simulink model "aerotest"  (R2021b)
settings: Solver=VariableStepAuto  StartTime=0.0  StopTime=10.0  RelTol=1e-3
undefined symbols (not defined in the file or in its folder): admireDB
libraries: simulink_extras x103, simulink x24, aerolibatmos2 x1
(part 10 of 13)

== system aerotest/RollMomentCoefficient/MachRegion1/Crmbeta/Crmbeta_ ==
  angleOfSideslip_deg : Inport
  angleOfAttack_deg : Inport  Port=2
  qacorr : Inport  Port=3
  mach_nd : Inport  Port=4
  Abs : Abs
  CRMBAL_BETA_ALFA : Lookup_n-D  BreakpointsForDimension1=admireDB.aerodata_asym_ext.CRMBAL.breakpoints.ALFA  BreakpointsForDimension2=admireDB.aerodata_asym_ext.CRMBAL.breakpoints.BETA  BreakpointsForDimension3=[5, 7]  Table=admireDB.aerodata_asym_ext.CRMBAL.newTable  ExtrapMethod=Clip  InternalRulePriority=Speed  RndMeth=Simplest  InputSameDT=on
      settings: InputPortMap=u0,u1
  CRMEB_QA_M : Lookup_n-D  BreakpointsForDimension1=admireDB.aerodata_asym_ext.CRMEB.breakpoints.M  BreakpointsForDimension2=admireDB.aerodata_asym_ext.CRMEB.breakpoints.QA  BreakpointsForDimension3=[5, 7]  Table=admireDB.aerodata_asym_ext.CRMEB.newTable  ExtrapMethod=Clip  InternalRulePriority=Speed  RndMeth=Simplest  InputSameDT=on
      settings: InputPortMap=u0,u1
  Degrees to Radians : simulink_extras/Transformations/Degrees to Radians
  Product : Product
  Product1 : Product
  Sign : Signum
  Sum : Sum  Inputs=|++
  Crmbeta : Outport
  wires:
  Sum/1 -> Crmbeta/1
  Product1/1 -> Sum/2
  Degrees to Radians/1 -> Product1/1
  CRMEB_QA_M/1 -> Product1/2
  Product/1 -> Sum/1
  Abs/1 -> CRMBAL_BETA_ALFA/2
  Sign/1 -> Product/1
  CRMBAL_BETA_ALFA/1 -> Product/2
  angleOfSideslip_deg/1 -> Abs/1, Sign/1, Degrees to Radians/1
  mach_nd/1 -> CRMEB_QA_M/1
  angleOfAttack_deg/1 -> CRMBAL_BETA_ALFA/1
  qacorr/1 -> CRMEB_QA_M/2

== system aerotest/RollMomentCoefficient/MachRegion1/Crmbetad/Crmbetad_ ==
  angleOfAttack_deg : Inport
  betad : Inport  Port=2
  CRMBDL_ALFA : Lookup_n-D  NumberOfTableDimensions=1  BreakpointsForDimension1=admireDB.aerodata_asym_ext.CRMBDL.breakpoints.ALFA  BreakpointsForDimension3=[5, 7]  Table=admireDB.aerodata_asym_ext.CRMBDL.newTable  ExtrapMethod=Clip  InternalRulePriority=Speed  RndMeth=Simplest  InputSameDT=on
  Product : Product  Inputs=**
  Crmbetad : Outport
  wires:
  angleOfAttack_deg/1 -> CRMBDL_ALFA/1
  Product/1 -> Crmbetad/1
  CRMBDL_ALFA/1 -> Product/1
  betad/1 -> Product/2

== system aerotest/RollMomentCoefficient/MachRegion1/Crmblg/Crmblg_ ==
  dLG : Inport
  angleOfAttack_deg : Inport  Port=2
  angleOfSideslip_deg : Inport  Port=3
  CRMBLST_NG_DOOR_ALFA : Lookup_n-D  BreakpointsForDimension1=admireDB.aerodata_asym_ext.CRMBLST.breakpoints.ALFA  BreakpointsForDimension2=admireDB.aerodata_asym_ext.CRMBLST.breakpoints.NG_DOOR  BreakpointsForDimension3=[5, 7]  Table=admireDB.aerodata_asym_ext.CRMBLST.newTable  ExtrapMethod=Clip  InternalRulePriority=Speed  RndMeth=Simplest  InputSameDT=on
      settings: InputPortMap=u0,u1
  Degrees to Radians : simulink_extras/Transformations/Degrees to Radians
  Product : Product  Inputs=3
  Crmblg : Outport
  wires:
  Degrees to Radians/1 -> Product/3
  CRMBLST_NG_DOOR_ALFA/1 -> Product/2
  dLG/1 -> CRMBLST_NG_DOOR_ALFA/2, Product/1
  angleOfAttack_deg/1 -> CRMBLST_NG_DOOR_ALFA/1
  Product/1 -> Crmblg/1
  angleOfSideslip_deg/1 -> Degrees to Radians/1

== system aerotest/RollMomentCoefficient/MachRegion1/Crmdai/Crmdai_ ==
  dAI : Inport
  angleOfAttack_deg : Inport  Port=2
  dEI : Inport  Port=3
  eieff : Inport  Port=4
  qacorr : Inport  Port=5
  mach_nd : Inport  Port=6
  Abs : Abs
  CRMDAAL_DA_ALFA : Lookup_n-D  BreakpointsForDimension1=admireDB.aerodata_asym_ext.CRMDAAL.breakpoints.ALFA  BreakpointsForDimension2=admireDB.aerodata_asym_ext.CRMDAAL.breakpoints.DA  BreakpointsForDimension3=[5, 7]  Table=admireDB.aerodata_asym_ext.CRMDAAL.newTable  ExtrapMethod=Clip  InternalRulePriority=Speed  RndMeth=Simplest  InputSameDT=on
      settings: InputPortMap=u0,u1
  CRMDAL_DE_ALFA : Lookup_n-D  BreakpointsForDimension1=admireDB.aerodata_asym_ext.CRMDAL.breakpoints.ALFA  BreakpointsForDimension2=admireDB.aerodata_asym_ext.CRMDAL.breakpoints.DE  BreakpointsForDimension3=[5, 7]  Table=admireDB.aerodata_asym_ext.CRMDAL.newTable  ExtrapMethod=Clip  InternalRulePriority=Speed  RndMeth=Simplest  InputSameDT=on
      settings: InputPortMap=u0,u1
  CRMDAL_DE_ALFA_1 : Lookup_n-D  BreakpointsForDimension1=admireDB.aerodata_asym_ext.CRMDAL.breakpoints.ALFA  BreakpointsForDimension2=admireDB.aerodata_asym_ext.CRMDAL.breakpoints.DE  BreakpointsForDimension3=[5, 7]  Table=admireDB.aerodata_asym_ext.CRMDAL.newTable  ExtrapMethod=Clip  InternalRulePriority=Speed  RndMeth=Simplest  InputSameDT=on
      settings: InputPortMap=u0,u1
  CRMEDAI_QA_M : Lookup_n-D  BreakpointsForDimension1=admireDB.aerodata_asym_ext.CRMEDAI.breakpoints.M  BreakpointsForDimension2=admireDB.aerodata_asym_ext.CRMEDAI.breakpoints.QA  BreakpointsForDimension3=[5, 7]  Table=admireDB.aerodata_asym_ext.CRMEDAI.newTable  ExtrapMethod=Clip  InternalRulePriority=Speed  RndMeth=Simplest  InputSameDT=on
      settings: InputPortMap=u0,u1
  Degrees to Radians : simulink_extras/Transformations/Degrees to Radians
  Product : Product
  Product1 : Product
  Product2 : Product  Inputs=3
  Sign : Signum
  Sum : Sum  Inputs=|+-
  Sum1 : Sum  Inputs=|++
  dE_cnst : Constant  Value=0.0
  Crmdai : Outport
  wires:
  CRMEDAI_QA_M/1 -> Product2/3
  qacorr/1 -> CRMEDAI_QA_M/2
  mach_nd/1 -> CRMEDAI_QA_M/1
  eieff/1 -> Product2/2
  Sum1/1 -> Product2/1
  Product/1 -> Sum1/2
  Product1/1 -> Sum1/1
  Sign/1 -> Product1/1
  CRMDAAL_DA_ALFA/1 -> Product1/2
  Degrees to Radians/1 -> Product/1
  Sum/1 -> Product/2
  CRMDAL_DE_ALFA_1/1 -> Sum/2
  CRMDAL_DE_ALFA/1 -> Sum/1
  dEI/1 -> CRMDAL_DE_ALFA/2
  dE_cnst/1 -> CRMDAL_DE_ALFA_1/2
  dAI/1 -> Abs/1, Sign/1, Degrees to Radians/1
  Abs/1 -> CRMDAAL_DA_ALFA/2
  angleOfAttack_deg/1 -> CRMDAAL_DA_ALFA/1, CRMDAL_DE_ALFA_1/1, CRMDAL_DE_ALFA/1
  Product2/1 -> Crmdai/1

== system aerotest/RollMomentCoefficient/MachRegion1/Crmdaib/Crmdaib_ ==
  angleOfAttack_deg : Inport
  dAI : Inport  Port=2
  angleOfSideslip_deg : Inport  Port=3
  eieff : Inport  Port=4
  Abs : Abs
  Abs1 : Abs
  Abs2 : Abs
  CRMDABAL_ALFA : Lookup_n-D  NumberOfTableDimensions=1  BreakpointsForDimension1=admireDB.aerodata_asym_ext.CRMDABAL.breakpoints.ALFA  BreakpointsForDimension3=[5, 7]  Table=admireDB.aerodata_asym_ext.CRMDABAL.newTable  ExtrapMethod=Clip  InternalRulePriority=Speed  RndMeth=Simplest  InputSameDT=on
  Constant : Constant  Value=30
  Constant1 : Constant  Value=20
  Product : Product  Inputs=**/*/*
  Crmdaib : Outport
  wires:
  eieff/1 -> Product/6
  Abs2/1 -> Product/4
  Constant1/1 -> Product/5
  angleOfSideslip_deg/1 -> Abs2/1
  Constant/1 -> Product/3
  Abs1/1 -> Product/2
  Abs/1 -> CRMDABAL_ALFA/1
  dAI/1 -> Abs1/1
  CRMDABAL_ALFA/1 -> Product/1
  angleOfAttack_deg/1 -> Abs/1
  Product/1 -> Crmdaib/1

== system aerotest/RollMomentCoefficient/MachRegion1/Crmday/Crmday_ ==
  dAY : Inport
  angleOfAttack_deg : Inport  Port=2
  dEY : Inport  Port=3
  eoeff : Inport  Port=4
  qacorr : Inport  Port=5
  mach_nd : Inport  Port=6
  Abs : Abs
  CRMDAAL_DA_ALFA : Lookup_n-D  BreakpointsForDimension1=admireDB.aerodata_asym_ext.CRMDAAL.breakpoints.ALFA  BreakpointsForDimension2=admireDB.aerodata_asym_ext.CRMDAAL.breakpoints.DA  BreakpointsForDimension3=[5, 7]  Table=admireDB.aerodata_asym_ext.CRMDAAL.newTable  ExtrapMethod=Clip  InternalRulePriority=Speed  RndMeth=Simplest  InputSameDT=on
      settings: InputPortMap=u0,u1
  CRMDAL_DE_ALFA : Lookup_n-D  BreakpointsForDimension1=admireDB.aerodata_asym_ext.CRMDAL.breakpoints.ALFA  BreakpointsForDimension2=admireDB.aerodata_asym_ext.CRMDAL.breakpoints.DE  BreakpointsForDimension3=[5, 7]  Table=admireDB.aerodata_asym_ext.CRMDAL.newTable  ExtrapMethod=Clip  InternalRulePriority=Speed  RndMeth=Simplest  InputSameDT=on
      settings: InputPortMap=u0,u1
  CRMDAL_DE_ALFA_1 : Lookup_n-D  BreakpointsForDimension1=admireDB.aerodata_asym_ext.CRMDAL.breakpoints.ALFA  BreakpointsForDimension2=admireDB.aerodata_asym_ext.CRMDAL.breakpoints.DE  BreakpointsForDimension3=[5, 7]  Table=admireDB.aerodata_asym_ext.CRMDAL.newTable  ExtrapMethod=Clip  InternalRulePriority=Speed  RndMeth=Simplest  InputSameDT=on
      settings: InputPortMap=u0,u1
  CRMEDAY_QA_M : Lookup_n-D  BreakpointsForDimension1=admireDB.aerodata_asym_ext.CRMEDAY.breakpoints.M  BreakpointsForDimension2=admireDB.aerodata_asym_ext.CRMEDAY.breakpoints.QA  BreakpointsForDimension3=[5, 7]  Table=admireDB.aerodata_asym_ext.CRMEDAY.newTable  ExtrapMethod=Clip  InternalRulePriority=Speed  RndMeth=Simplest  InputSameDT=on
      settings: InputPortMap=u0,u1
  Degrees to Radians : simulink_extras/Transformations/Degrees to Radians
  Product : Product
  Product1 : Product
  Product2 : Product  Inputs=3
  Sign : Signum
  Sum : Sum  Inputs=|+-
  Sum1 : Sum  Inputs=|++
  dE_cnst : Constant  Value=0.0
  Crmdai : Outport
  wires:
  dE_cnst/1 -> CRMDAL_DE_ALFA_1/2
  Product2/1 -> Crmdai/1
  angleOfAttack_deg/1 -> CRMDAL_DE_ALFA_1/1, CRMDAL_DE_ALFA/1, CRMDAAL_DA_ALFA/1
  Abs/1 -> CRMDAAL_DA_ALFA/2
  dAY/1 -> Abs/1, Sign/1, Degrees to Radians/1
  dEY/1 -> CRMDAL_DE_ALFA/2
  CRMDAL_DE_ALFA/1 -> Sum/1
  CRMDAL_DE_ALFA_1/1 -> Sum/2
  Sum/1 -> Product/2
  Degrees to Radians/1 -> Product/1
  CRMDAAL_DA_ALFA/1 -> Product1/2
  Sign/1 -> Product1/1
  Product1/1 -> Sum1/1
  Product/1 -> Sum1/2
  Sum1/1 -> Product2/1
  eoeff/1 -> Product2/2
  qacorr/1 -> CRMEDAY_QA_M/2
  mach_nd/1 -> CRMEDAY_QA_M/1
  CRMEDAY_QA_M/1 -> Product2/3

== system aerotest/RollMomentCoefficient/MachRegion1/Crmdayb/Crmdaib_ ==
  angleOfAttack_deg : Inport
  dAY : Inport  Port=2
  angleOfSideslip_deg : Inport  Port=3
  eoeff : Inport  Port=4
  Abs : Abs
  Abs1 : Abs
  Abs2 : Abs
  CRMDABAL_ALFA : Lookup_n-D  NumberOfTableDimensions=1  BreakpointsForDimension1=admireDB.aerodata_asym_ext.CRMDABAL.breakpoints.ALFA  BreakpointsForDimension3=[5, 7]  Table=admireDB.aerodata_asym_ext.CRMDABAL.newTable  ExtrapMethod=Clip  InternalRulePriority=Speed  RndMeth=Simplest  InputSameDT=on
  Constant : Constant  Value=30
  Constant1 : Constant  Value=20
  Product : Product  Inputs=**/*/*
  Crmdaib : Outport
  wires:
  Product/1 -> Crmdaib/1
  angleOfAttack_deg/1 -> Abs/1
  CRMDABAL_ALFA/1 -> Product/1
  dAY/1 -> Abs1/1
  Abs/1 -> CRMDABAL_ALFA/1
  Abs1/1 -> Product/2
  Constant/1 -> Product/3
  angleOfSideslip_deg/1 -> Abs2/1
  Constant1/1 -> Product/5
  Abs2/1 -> Product/4
  eoeff/1 -> Product/6

== system aerotest/RollMomentCoefficient/MachRegion1/Crmdna/Crmdna_ ==
  dNE : Inport
  angleOfAttack_deg : Inport  Port=2
  dNA : Inport  Port=3
  CRMDNAAL_DNE_ALFA : Lookup_n-D  BreakpointsForDimension1=admireDB.aerodata_asym_ext.CRMDNAAL.breakpoints.ALFA  BreakpointsForDimension2=admireDB.aerodata_asym_ext.CRMDNAAL.breakpoints.DNE  BreakpointsForDimension3=[5, 7]  Table=admireDB.aerodata_asym_ext.CRMDNAAL.newTable  ExtrapMethod=Clip  InternalRulePriority=Speed  RndMeth=Simplest  InputSameDT=on
      settings: InputPortMap=u0,u1
  Degrees to Radians : simulink_extras/Transformations/Degrees to Radians
  Product : Product  Inputs=**
  Crmdna : Outport
  wires:
  Degrees to Radians/1 -> Product/2
  CRMDNAAL_DNE_ALFA/1 -> Product/1
  dNA/1 -> Degrees to Radians/1
  angleOfAttack_deg/1 -> CRMDNAAL_DNE_ALFA/1
  dNE/1 -> CRMDNAAL_DNE_ALFA/2
  Product/1 -> Crmdna/1

== system aerotest/RollMomentCoefficient/MachRegion1/Crmdr/Crmdr_ ==
  angleOfAttack_deg : Inport
  dR : Inport  Port=2
  angleOfSideslip_deg : Inport  Port=3
  qacorr : Inport  Port=4
  mach_nd : Inport  Port=5
  Abs : Abs
  CRMBDRAL_ALFA_DR_BETA : Lookup_n-D  NumberOfTableDimensions=3  BreakpointsForDimension1=admireDB.aerodata_asym_ext.CRMBDRAL.breakpoints.ALFA  BreakpointsForDimension2=admireDB.aerodata_asym_ext.CRMBDRAL.breakpoints.DR  BreakpointsForDimension3=admireDB.aerodata_asym_ext.CRMBDRAL.breakpoints.BETA  Table=admireDB.aerodata_asym_ext.CRMBDRAL.newTable  ExtrapMethod=Clip  InternalRulePriority=Speed  RndMeth=Simplest  InputSameDT=on
      settings: InputPortMap=u0,u1,u2
  CRMEDR_QA_M : Lookup_n-D  BreakpointsForDimension1=admireDB.aerodata_asym_ext.CRMEDR.breakpoints.M  BreakpointsForDimension2=admireDB.aerodata_asym_ext.CRMEDR.breakpoints.QA  BreakpointsForDimension3=[5, 7]  Table=admireDB.aerodata_asym_ext.CRMEDR.newTable  ExtrapMethod=Clip  InternalRulePriority=Speed  RndMeth=Simplest  InputSameDT=on
      settings: InputPortMap=u0,u1
  Product : Product
  Crmdr : Outport
  wires:
  CRMBDRAL_ALFA_DR_BETA/1 -> Product/1
  CRMEDR_QA_M/1 -> Product/2
  angleOfAttack_deg/1 -> CRMBDRAL_ALFA_DR_BETA/1
  angleOfSideslip_deg/1 -> Abs/1
  dR/1 -> CRMBDRAL_ALFA_DR_BETA/2
  Abs/1 -> CRMBDRAL_ALFA_DR_BETA/3
  qacorr/1 -> CRMEDR_QA_M/2
  mach_nd/1 -> CRMEDR_QA_M/1
  Product/1 -> Crmdr/1

== system aerotest/RollMomentCoefficient/MachRegion1/Crmp/Crmp_ ==
  dN : Inport
  angleOfAttack_deg : Inport  Port=2
  qacorr : Inport  Port=3
  mach_nd : Inport  Port=4
  pc : Inport  Port=5
  CRMEP_QA_M : Lookup_n-D  BreakpointsForDimension1=admireDB.aerodata_asym_ext.CRMEP.breakpoints.M  BreakpointsForDimension2=admireDB.aerodata_asym_ext.CRMEP.breakpoints.QA  BreakpointsForDimension3=[5, 7]  Table=admireDB.aerodata_asym_ext.CRMEP.newTable  ExtrapMethod=Clip  InternalRulePriority=Speed  RndMeth=Simplest  InputSameDT=on
      settings: InputPortMap=u0,u1
  CRMPAL_DN_ALFA : Lookup_n-D  BreakpointsForDimension1=admireDB.aerodata_asym_ext.CRMPAL.breakpoints.ALFA  BreakpointsForDimension2=admireDB.aerodata_asym_ext.CRMPAL.breakpoints.DN  BreakpointsForDimension3=[5, 7]  Table=admireDB.aerodata_asym_ext.CRMPAL.newTable  ExtrapMethod=Clip  InternalRulePriority=Speed  RndMeth=Simplest  InputSameDT=on
      settings: InputPortMap=u0,u1
  Product : Product  Inputs=3
  Crmp : Outport
  wires:
  Product/1 -> Crmp/1
  pc/1 -> Product/2
  CRMEP_QA_M/1 -> Product/3
  CRMPAL_DN_ALFA/1 -> Product/1
  angleOfAttack_deg/1 -> CRMPAL_DN_ALFA/1
  dN/1 -> CRMPAL_DN_ALFA/2
  mach_nd/1 -> CRMEP_QA_M/1
  qacorr/1 -> CRMEP_QA_M/2

== system aerotest/RollMomentCoefficient/MachRegion1/Crmpbeta/Crmpbeta_ ==
  angleOfSideslip_deg : Inport
  angleOfAttack_deg : Inport  Port=2
  pc : Inport  Port=3
  Abs : Abs
  CRMPBA_BETA_ALFA : Lookup_n-D  BreakpointsForDimension1=admireDB.aerodata_asym_ext.CRMPBA.breakpoints.ALFA  BreakpointsForDimension2=admireDB.aerodata_asym_ext.CRMPBA.breakpoints.BETA  BreakpointsForDimension3=[5, 7]  Table=admireDB.aerodata_asym_ext.CRMPBA.newTable  ExtrapMethod=Clip  InternalRulePriority=Speed  RndMeth=Simplest  InputSameDT=on
      settings: InputPortMap=u0,u1
  Product : Product  Inputs=**
  Crmpbeta : Outport
  wires:
  Abs/1 -> CRMPBA_BETA_ALFA/2
  CRMPBA_BETA_ALFA/1 -> Product/1
  angleOfSideslip_deg/1 -> Abs/1
  angleOfAttack_deg/1 -> CRMPBA_BETA_ALFA/1
  pc/1 -> Product/2
  Product/1 -> Crmpbeta/1

== system aerotest/RollMomentCoefficient/MachRegion1/Crmr/Crmr_ ==
  dN : Inport
  angleOfAttack_deg : Inport  Port=2
  rc : Inport  Port=3
  CRMRAL_DN_ALFA : Lookup_n-D  BreakpointsForDimension1=admireDB.aerodata_asym_ext.CRMRAL.breakpoints.ALFA  BreakpointsForDimension2=admireDB.aerodata_asym_ext.CRMRAL.breakpoints.DN  BreakpointsForDimension3=[5, 7]  Table=admireDB.aerodata_asym_ext.CRMRAL.newTable  ExtrapMethod=Clip  InternalRulePriority=Speed  RndMeth=Simplest  InputSameDT=on
      settings: InputPortMap=u0,u1
  Product : Product  Inputs=**
  Crmr : Outport
  wires:
  CRMRAL_DN_ALFA/1 -> Product/1
  angleOfAttack_deg/1 -> CRMRAL_DN_ALFA/1
  dN/1 -> CRMRAL_DN_ALFA/2
  Product/1 -> Crmr/1
  rc/1 -> Product/2

== system aerotest/RollMomentCoefficient/MachRegion1/Crmrbeta/Crmrbeta_ ==
  angleOfSideslip_deg : Inport
  angleOfAttack_deg : Inport  Port=2
  rc : Inport  Port=3
  Abs : Abs
  CRMRBA_BETA_ALFA : Lookup_n-D  BreakpointsForDimension1=admireDB.aerodata_asym_ext.CRMRBA.breakpoints.ALFA  BreakpointsForDimension2=admireDB.aerodata_asym_ext.CRMRBA.breakpoints.BETA  BreakpointsForDimension3=[5, 7]  Table=admireDB.aerodata_asym_ext.CRMRBA.newTable  ExtrapMethod=Clip  InternalRulePriority=Speed  RndMeth=Simplest  InputSameDT=on
      settings: InputPortMap=u0,u1
  Product : Product  Inputs=**
  Crmrbeta : Outport
  wires:
  Abs/1 -> CRMRBA_BETA_ALFA/2
  angleOfSideslip_deg/1 -> Abs/1
  angleOfAttack_deg/1 -> CRMRBA_BETA_ALFA/1
  rc/1 -> Product/2
  Product/1 -> Crmrbeta/1
  CRMRBA_BETA_ALFA/1 -> Product/1

== system aerotest/RollMomentCoefficient/MachRegion1/Crmrde/Crmrde_ ==
  mach_nd : Inport
  angleOfAttack_deg : Inport  Port=2
  rc : Inport  Port=3
  dEI : Inport  Port=4
  eieff : Inport  Port=5
  dey : Inport  Port=6
  eoeff : Inport  Port=7
  CRMRDEM_M : Lookup_n-D  NumberOfTableDimensions=1  BreakpointsForDimension1=admireDB.aerodata_asym_ext.CRMRDEM.breakpoints.M  BreakpointsForDimension3=[5, 7]  Table=admireDB.aerodata_asym_ext.CRMRDEM.newTable  ExtrapMethod=Clip  InternalRulePriority=Speed  RndMeth=Simplest  InputSameDT=on
  CRMRKA_ALFA : Lookup_n-D  NumberOfTableDimensions=1  BreakpointsForDimension1=admireDB.aerodata_asym_ext.CRMRKA.breakpoints.ALFA  BreakpointsForDimension3=[5, 7]  Table=admireDB.aerodata_asym_ext.CRMRKA.newTable  ExtrapMethod=Clip  InternalRulePriority=Speed  RndMeth=Simplest  InputSameDT=on
  Constant : Constant  Value=1/30
  Constant1 : Constant  Value=1/30
  Product : Product  Inputs=****
  Product1 : Product  Inputs=3
  Product2 : Product  Inputs=3
  Sum : Sum  Inputs=|++
  Crmrbeta : Outport
  wires:
  Sum/1 -> Product/4
  Product2/1 -> Sum/2
  Product1/1 -> Sum/1
  dey/1 -> Product2/1
  eoeff/1 -> Product2/3
  Constant1/1 -> Product2/2
  Constant/1 -> Product1/2
  eieff/1 -> Product1/3
  dEI/1 -> Product1/1
  CRMRKA_ALFA/1 -> Product/2
  CRMRDEM_M/1 -> Product/1
  mach_nd/1 -> CRMRDEM_M/1
  angleOfAttack_deg/1 -> CRMRKA_ALFA/1
  Product/1 -> Crmrbeta/1
  rc/1 -> Product/3

== system aerotest/RollMomentCoefficient/MachRegion2/Crmbasic/Crmbasic_ ==
  angleOfAttack_deg : Inport
  tflow : Inport  Port=2
  Abs : Abs
  CRMZERO_ALFA : Lookup_n-D  NumberOfTableDimensions=1  BreakpointsForDimension1=admireDB.aerodata_asym_ext.CRMZERO.breakpoints.ALFA  BreakpointsForDimension3=[5, 7]  Table=admireDB.aerodata_asym_ext.CRMZERO.newTable  ExtrapMethod=Clip  InternalRulePriority=Speed  RndMeth=Simplest  InputSameDT=on
  Product : Product
  Crmbasic : Outport
  wires:
  tflow/1 -> Product/2
  Product/1 -> Crmbasic/1
  CRMZERO_ALFA/1 -> Product/1
  angleOfAttack_deg/1 -> Abs/1
  Abs/1 -> CRMZERO_ALFA/1

== system aerotest/RollMomentCoefficient/MachRegion2/Crmbde/Crmbde_ ==
  angleOfAttack_deg : Inport
  dN : Inport  Port=2
  dEI : Inport  Port=3
  angleOfSideslip_deg : Inport  Port=4
  dEY : Inport  Port=5
  eieff : Inport  Port=6
  eoeff : Inport  Port=7
  Abs : Abs
  CRMDEB_ALFA_DN_DE_BETA : Lookup_n-D  NumberOfTableDimensions=4  BreakpointsForDimension1=admireDB.aerodata_asym_ext.CRMDEB.breakpoints.ALFA  BreakpointsForDimension2=admireDB.aerodata_asym_ext.CRMDEB.breakpoints.DN  BreakpointsForDimension3=admireDB.aerodata_asym_ext.CRMDEB.breakpoints.DE  BreakpointsForDimension4=admireDB.aerodata_asym_ext.CRMDEB.breakpoints.BETA  Table=admireDB.aerodata_asym_ext.CRMDEB.newTable  ExtrapMethod=Clip  InternalRulePriority=Speed  RndMeth=Simplest  InputSameDT=on
      settings: InputPortMap=u0,u1,u2,u3
  CRMDEB_ALFA_DN_DE_BETA1 : Lookup_n-D  NumberOfTableDimensions=4  BreakpointsForDimension1=admireDB.aerodata_asym_ext.CRMDEB.breakpoints.ALFA  BreakpointsForDimension2=admireDB.aerodata_asym_ext.CRMDEB.breakpoints.DN  BreakpointsForDimension3=admireDB.aerodata_asym_ext.CRMDEB.breakpoints.DE  BreakpointsForDimension4=admireDB.aerodata_asym_ext.CRMDEB.breakpoints.BETA  Table=admireDB.aerodata_asym_ext.CRMDEB.newTable  ExtrapMethod=Clip  InternalRulePriority=Speed  RndMeth=Simplest  InputSameDT=on
      settings: InputPortMap=u0,u1,u2,u3
  Product : Product  Inputs=**
  Product1 : Product  Inputs=**
  Product2 : Product
  Sign : Signum
  Sum : Sum  Inputs=|++
  Crmbde : Outport
  wires:
  dEY/1 -> CRMDEB_ALFA_DN_DE_BETA1/3
  dEI/1 -> CRMDEB_ALFA_DN_DE_BETA/3
  dN/1 -> CRMDEB_ALFA_DN_DE_BETA/2, CRMDEB_ALFA_DN_DE_BETA1/2
  angleOfAttack_deg/1 -> CRMDEB_ALFA_DN_DE_BETA/1, CRMDEB_ALFA_DN_DE_BETA1/1
  Abs/1 -> CRMDEB_ALFA_DN_DE_BETA1/4, CRMDEB_ALFA_DN_DE_BETA/4
  angleOfSideslip_deg/1 -> Sign/1, Abs/1
  CRMDEB_ALFA_DN_DE_BETA/1 -> Product/1
  CRMDEB_ALFA_DN_DE_BETA1/1 -> Product1/2
  eieff/1 -> Product/2
  eoeff/1 -> Product1/1
  Sum/1 -> Product2/2
  Product/1 -> Sum/1
  Product1/1 -> Sum/2
  Product2/1 -> Crmbde/1
  Sign/1 -> Product2/1

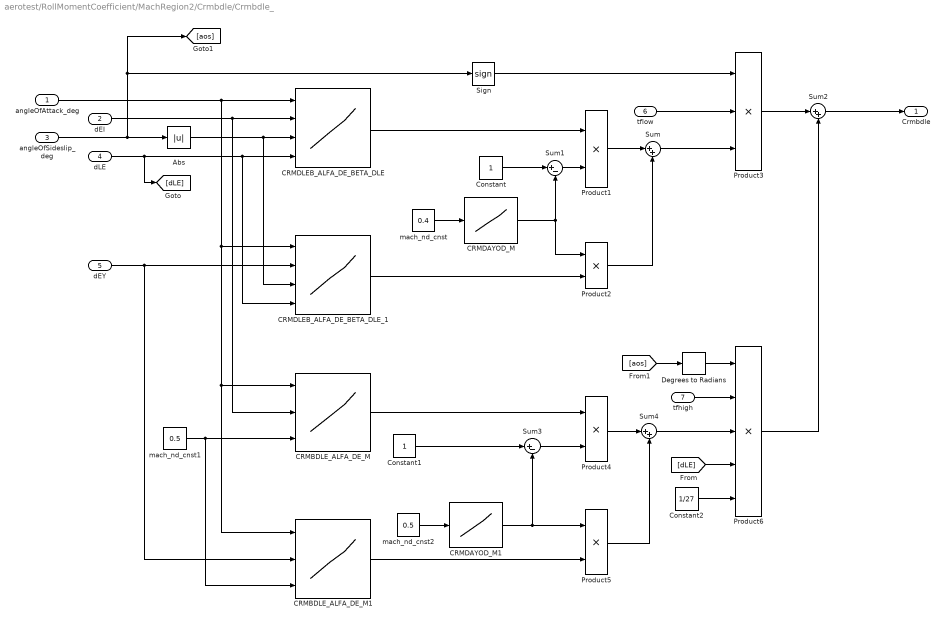
== system aerotest/RollMomentCoefficient/MachRegion2/Crmbdle/Crmbdle_ ==
  angleOfAttack_deg : Inport
  dEI : Inport  Port=2
  angleOfSideslip_deg : Inport  Port=3
  dLE : Inport  Port=4
  dEY : Inport  Port=5
  tflow : Inport  Port=6
  tfhigh : Inport  Port=7
  Abs : Abs
  CRMBDLE_ALFA_DE_M : Lookup_n-D  NumberOfTableDimensions=3  BreakpointsForDimension1=admireDB.aerodata_asym_ext.CRMBDLE.breakpoints.ALFA  BreakpointsForDimension2=admireDB.aerodata_asym_ext.CRMBDLE.breakpoints.DE  BreakpointsForDimension3=admireDB.aerodata_asym_ext.CRMBDLE.breakpoints.M  Table=admireDB.aerodata_asym_ext.CRMBDLE.newTable  ExtrapMethod=Clip  InternalRulePriority=Speed  RndMeth=Simplest  InputSameDT=on
      settings: InputPortMap=u0,u1,u2
  CRMBDLE_ALFA_DE_M1 : Lookup_n-D  NumberOfTableDimensions=3  BreakpointsForDimension1=admireDB.aerodata_asym_ext.CRMBDLE.breakpoints.ALFA  BreakpointsForDimension2=admireDB.aerodata_asym_ext.CRMBDLE.breakpoints.DE  BreakpointsForDimension3=admireDB.aerodata_asym_ext.CRMBDLE.breakpoints.M  Table=admireDB.aerodata_asym_ext.CRMBDLE.newTable  ExtrapMethod=Clip  InternalRulePriority=Speed  RndMeth=Simplest  InputSameDT=on
      settings: InputPortMap=u0,u1,u2
  CRMDAYOD_M : Lookup_n-D  NumberOfTableDimensions=1  BreakpointsForDimension1=admireDB.aerodata_asym_ext.CRMDAYOD.breakpoints.M  BreakpointsForDimension3=[5, 7]  Table=admireDB.aerodata_asym_ext.CRMDAYOD.newTable  ExtrapMethod=Clip  InternalRulePriority=Speed  RndMeth=Simplest  InputSameDT=on
  CRMDAYOD_M1 : Lookup_n-D  NumberOfTableDimensions=1  BreakpointsForDimension1=admireDB.aerodata_asym_ext.CRMDAYOD.breakpoints.M  BreakpointsForDimension3=[5, 7]  Table=admireDB.aerodata_asym_ext.CRMDAYOD.newTable  ExtrapMethod=Clip  InternalRulePriority=Speed  RndMeth=Simplest  InputSameDT=on
  CRMDLEB_ALFA_DE_BETA_DLE : Lookup_n-D  NumberOfTableDimensions=4  BreakpointsForDimension1=admireDB.aerodata_asym_ext.CRMDLEB.breakpoints.ALFA  BreakpointsForDimension2=admireDB.aerodata_asym_ext.CRMDLEB.breakpoints.DE  BreakpointsForDimension3=admireDB.aerodata_asym_ext.CRMDLEB.breakpoints.BETA  BreakpointsForDimension4=admireDB.aerodata_asym_ext.CRMDLEB.breakpoints.DLE  Table=admireDB.aerodata_asym_ext.CRMDLEB.newTable  ExtrapMethod=Clip  InternalRulePriority=Speed  RndMeth=Simplest  InputSameDT=on
      settings: InputPortMap=u0,u1,u2,u3
  CRMDLEB_ALFA_DE_BETA_DLE_1 : Lookup_n-D  NumberOfTableDimensions=4  BreakpointsForDimension1=admireDB.aerodata_asym_ext.CRMDLEB.breakpoints.ALFA  BreakpointsForDimension2=admireDB.aerodata_asym_ext.CRMDLEB.breakpoints.DE  BreakpointsForDimension3=admireDB.aerodata_asym_ext.CRMDLEB.breakpoints.BETA  BreakpointsForDimension4=admireDB.aerodata_asym_ext.CRMDLEB.breakpoints.DLE  Table=admireDB.aerodata_asym_ext.CRMDLEB.newTable  ExtrapMethod=Clip  InternalRulePriority=Speed  RndMeth=Simplest  InputSameDT=on
      settings: InputPortMap=u0,u1,u2,u3
  Constant : Constant
  Constant1 : Constant
  Constant2 : Constant  Value=1/27
  Degrees to Radians : simulink_extras/Transformations/Degrees to Radians
  Product1 : Product
  Product2 : Product  Inputs=**
  Product3 : Product  Inputs=3
  Product4 : Product  Inputs=**
  Product5 : Product  Inputs=**
  Product6 : Product  Inputs=5
  Sign : Signum
  Sum : Sum  Inputs=|++
  Sum1 : Sum  Inputs=|+-
  Sum2 : Sum  Inputs=|++
  Sum3 : Sum  Inputs=|+-
  Sum4 : Sum  Inputs=|++
  mach_nd_cnst : Constant  Value=0.4
  mach_nd_cnst1 : Constant  Value=0.5
  mach_nd_cnst2 : Constant  Value=0.5
  Crmbdle : Outport
  wires:
  mach_nd_cnst1/1 -> CRMBDLE_ALFA_DE_M1/3, CRMBDLE_ALFA_DE_M/3
  angleOfAttack_deg/1 -> CRMDLEB_ALFA_DE_BETA_DLE/1, CRMDLEB_ALFA_DE_BETA_DLE_1/1, CRMBDLE_ALFA_DE_M1/1, CRMBDLE_ALFA_DE_M/1
  Sum2/1 -> Crmbdle/1
  Product6/1 -> Sum2/2
  Constant2/1 -> Product6/5
  Degrees to Radians/1 -> Product6/1
  tfhigh/1 -> Product6/2
  [dLE] -> Product6/4
  [aos] -> Degrees to Radians/1
  Sum4/1 -> Product6/3
  Product5/1 -> Sum4/2
  CRMBDLE_ALFA_DE_M1/1 -> Product5/2
  Product4/1 -> Sum4/1
  Sum3/1 -> Product4/2
  CRMBDLE_ALFA_DE_M/1 -> Product4/1
  Constant1/1 -> Sum3/1
  CRMDAYOD_M1/1 -> Product5/1, Sum3/2
  mach_nd_cnst2/1 -> CRMDAYOD_M1/1
  dEI/1 -> CRMDLEB_ALFA_DE_BETA_DLE/2, CRMBDLE_ALFA_DE_M/2
  tflow/1 -> Product3/2
  Sum/1 -> Product3/3
  Product2/1 -> Sum/2
  Product1/1 -> Sum/1
  Sum1/1 -> Product1/2
  mach_nd_cnst/1 -> CRMDAYOD_M/1
  CRMDAYOD_M/1 -> Sum1/2, Product2/1
  Constant/1 -> Sum1/1
  Product3/1 -> Sum2/1
  dEY/1 -> CRMBDLE_ALFA_DE_M1/2, CRMDLEB_ALFA_DE_BETA_DLE_1/2
  angleOfSideslip_deg/1 -> [aos], Sign/1, Abs/1
  dLE/1 -> CRMDLEB_ALFA_DE_BETA_DLE_1/4, CRMDLEB_ALFA_DE_BETA_DLE/4, [dLE]
  Abs/1 -> CRMDLEB_ALFA_DE_BETA_DLE_1/3, CRMDLEB_ALFA_DE_BETA_DLE/3
  Sign/1 -> Product3/1
  CRMDLEB_ALFA_DE_BETA_DLE_1/1 -> Product2/2
  CRMDLEB_ALFA_DE_BETA_DLE/1 -> Product1/1

== system aerotest/RollMomentCoefficient/MachRegion2/Crmbdn/Crmbdn_ ==
  angleOfSideslip_deg : Inport
  dN : Inport  Port=2
  angleOfAttack_deg : Inport  Port=3
  tflow : Inport  Port=4
  tfhigh : Inport  Port=5
  Abs : Abs
  CRMBMDN_DN_M : Lookup_n-D  BreakpointsForDimension1=admireDB.aerodata_asym_ext.CRMBMDN.breakpoints.M  BreakpointsForDimension2=admireDB.aerodata_asym_ext.CRMBMDN.breakpoints.DN  BreakpointsForDimension3=[5, 7]  Table=admireDB.aerodata_asym_ext.CRMBMDN.newTable  ExtrapMethod=Clip  InternalRulePriority=Speed  RndMeth=Simplest  InputSameDT=on
      settings: InputPortMap=u0,u1
  CRMDNB_ALFA_DN_BETA : Lookup_n-D  NumberOfTableDimensions=3  BreakpointsForDimension1=admireDB.aerodata_asym_ext.CRMDNB.breakpoints.ALFA  BreakpointsForDimension2=admireDB.aerodata_asym_ext.CRMDNB.breakpoints.DN  BreakpointsForDimension3=admireDB.aerodata_asym_ext.CRMDNB.breakpoints.BETA  Table=admireDB.aerodata_asym_ext.CRMDNB.newTable  ExtrapMethod=Clip  InternalRulePriority=Speed  RndMeth=Simplest  InputSameDT=on
      settings: InputPortMap=u0,u1,u2
  Degrees to Radians : simulink_extras/Transformations/Degrees to Radians
  Product : Product  Inputs=3
  Product1 : Product  Inputs=***
  Sign : Signum
  Sum : Sum  Inputs=|++
  mach_nd_cnst : Constant  Value=0.5
  Crmbdn : Outport
  wires:
  angleOfAttack_deg/1 -> CRMDNB_ALFA_DN_BETA/1
  Abs/1 -> CRMDNB_ALFA_DN_BETA/3
  Sum/1 -> Crmbdn/1
  Product1/1 -> Sum/2
  tfhigh/1 -> Product1/2
  Degrees to Radians/1 -> Product1/3
  CRMBMDN_DN_M/1 -> Product1/1
  mach_nd_cnst/1 -> CRMBMDN_DN_M/1
  angleOfSideslip_deg/1 -> Sign/1, Degrees to Radians/1, Abs/1
  dN/1 -> CRMBMDN_DN_M/2, CRMDNB_ALFA_DN_BETA/2
  tflow/1 -> Product/2
  Product/1 -> Sum/1
  CRMDNB_ALFA_DN_BETA/1 -> Product/3
  Sign/1 -> Product/1

== system aerotest/RollMomentCoefficient/MachRegion2/Crmbeta/Crmbeta_ ==
  angleOfSideslip_deg : Inport
  angleOfAttack_deg : Inport  Port=2
  tflow : Inport  Port=3
  thigh : Inport  Port=4
  qacorr : Inport  Port=5
  mach_nd : Inport  Port=6
  Abs : Abs
  CRMBAL_BETA_ALFA : Lookup_n-D  BreakpointsForDimension1=admireDB.aerodata_asym_ext.CRMBAL.breakpoints.ALFA  BreakpointsForDimension2=admireDB.aerodata_asym_ext.CRMBAL.breakpoints.BETA  BreakpointsForDimension3=[5, 7]  Table=admireDB.aerodata_asym_ext.CRMBAL.newTable  ExtrapMethod=Clip  InternalRulePriority=Speed  RndMeth=Simplest  InputSameDT=on
      settings: InputPortMap=u0,u1
  CRMBMA_M_ALFA : Lookup_n-D  BreakpointsForDimension1=admireDB.aerodata_asym_ext.CRMBMA.breakpoints.ALFA  BreakpointsForDimension2=admireDB.aerodata_asym_ext.CRMBMA.breakpoints.M  BreakpointsForDimension3=[5, 7]  Table=admireDB.aerodata_asym_ext.CRMBMA.newTable  ExtrapMethod=Clip  InternalRulePriority=Speed  RndMeth=Simplest  InputSameDT=on
      settings: InputPortMap=u0,u1
  CRMEB_QA_M : Lookup_n-D  BreakpointsForDimension1=admireDB.aerodata_asym_ext.CRMEB.breakpoints.M  BreakpointsForDimension2=admireDB.aerodata_asym_ext.CRMEB.breakpoints.QA  BreakpointsForDimension3=[5, 7]  Table=admireDB.aerodata_asym_ext.CRMEB.newTable  ExtrapMethod=Clip  InternalRulePriority=Speed  RndMeth=Simplest  InputSameDT=on
      settings: InputPortMap=u0,u1
  Degrees to Radians : simulink_extras/Transformations/Degrees to Radians
  Product : Product  Inputs=3
  Product1 : Product
  Product2 : Product  Inputs=3
  Sign : Signum
  Sum : Sum  Inputs=+++
  mach_nd_cnst : Constant  Value=0.5
  Crmbeta : Outport
  wires:
  Product2/1 -> Sum/2
  thigh/1 -> Product2/1
  CRMBMA_M_ALFA/1 -> Product2/2
  mach_nd_cnst/1 -> CRMBMA_M_ALFA/2
  angleOfAttack_deg/1 -> CRMBAL_BETA_ALFA/1, CRMBMA_M_ALFA/1
  tflow/1 -> Product/3
  qacorr/1 -> CRMEB_QA_M/2
  mach_nd/1 -> CRMEB_QA_M/1
  angleOfSideslip_deg/1 -> Abs/1, Sign/1, Degrees to Radians/1
  CRMBAL_BETA_ALFA/1 -> Product/2
  Sign/1 -> Product/1
  Abs/1 -> CRMBAL_BETA_ALFA/2
  Product/1 -> Sum/1
  CRMEB_QA_M/1 -> Product1/2
  Degrees to Radians/1 -> Product1/1, Product2/3
  Product1/1 -> Sum/3
  Sum/1 -> Crmbeta/1

== system aerotest/RollMomentCoefficient/MachRegion2/Crmbetad/Crmbetad_ ==
  angleOfAttack_deg : Inport
  betad : Inport  Port=2
  tflow : Inport  Port=3
  tfhigh : Inport  Port=4
  CRMBDH_ALFA_M : Lookup_n-D  BreakpointsForDimension1=admireDB.aerodata_asym_ext.CRMBDH.breakpoints.M  BreakpointsForDimension2=admireDB.aerodata_asym_ext.CRMBDH.breakpoints.ALFA  BreakpointsForDimension3=[5, 7]  Table=admireDB.aerodata_asym_ext.CRMBDH.newTable  ExtrapMethod=Clip  InternalRulePriority=Speed  RndMeth=Simplest  InputSameDT=on
      settings: InputPortMap=u0,u1
  CRMBDL_ALFA : Lookup_n-D  NumberOfTableDimensions=1  BreakpointsForDimension1=admireDB.aerodata_asym_ext.CRMBDL.breakpoints.ALFA  BreakpointsForDimension3=[5, 7]  Table=admireDB.aerodata_asym_ext.CRMBDL.newTable  ExtrapMethod=Clip  InternalRulePriority=Speed  RndMeth=Simplest  InputSameDT=on
  Product : Product  Inputs=**
  Product1 : Product  Inputs=**
  Product2 : Product  Inputs=**
  Sum : Sum  Inputs=|++
  mach_nd_cnst : Constant  Value=0.5
  Crmbetad : Outport
  wires:
  Sum/1 -> Product/1
  Product1/1 -> Sum/1
  Product2/1 -> Sum/2
  tfhigh/1 -> Product2/1
  tflow/1 -> Product1/2
  CRMBDH_ALFA_M/1 -> Product2/2
  mach_nd_cnst/1 -> CRMBDH_ALFA_M/1
  betad/1 -> Product/2
  CRMBDL_ALFA/1 -> Product1/1
  Product/1 -> Crmbetad/1
  angleOfAttack_deg/1 -> CRMBDL_ALFA/1, CRMBDH_ALFA_M/2

== system aerotest/RollMomentCoefficient/MachRegion2/Crmblg/Crmblg_ ==
  dLG : Inport
  angleOfAttack_deg : Inport  Port=2
  angleOfSideslip_deg : Inport  Port=3
  CRMBLST_NG_DOOR_ALFA : Lookup_n-D  BreakpointsForDimension1=admireDB.aerodata_asym_ext.CRMBLST.breakpoints.ALFA  BreakpointsForDimension2=admireDB.aerodata_asym_ext.CRMBLST.breakpoints.NG_DOOR  BreakpointsForDimension3=[5, 7]  Table=admireDB.aerodata_asym_ext.CRMBLST.newTable  ExtrapMethod=Clip  InternalRulePriority=Speed  RndMeth=Simplest  InputSameDT=on
      settings: InputPortMap=u0,u1
  Degrees to Radians : simulink_extras/Transformations/Degrees to Radians
  Product : Product  Inputs=3
  Crmblg : Outport
  wires:
  angleOfSideslip_deg/1 -> Degrees to Radians/1
  Product/1 -> Crmblg/1
  angleOfAttack_deg/1 -> CRMBLST_NG_DOOR_ALFA/1
  dLG/1 -> CRMBLST_NG_DOOR_ALFA/2, Product/1
  CRMBLST_NG_DOOR_ALFA/1 -> Product/2
  Degrees to Radians/1 -> Product/3

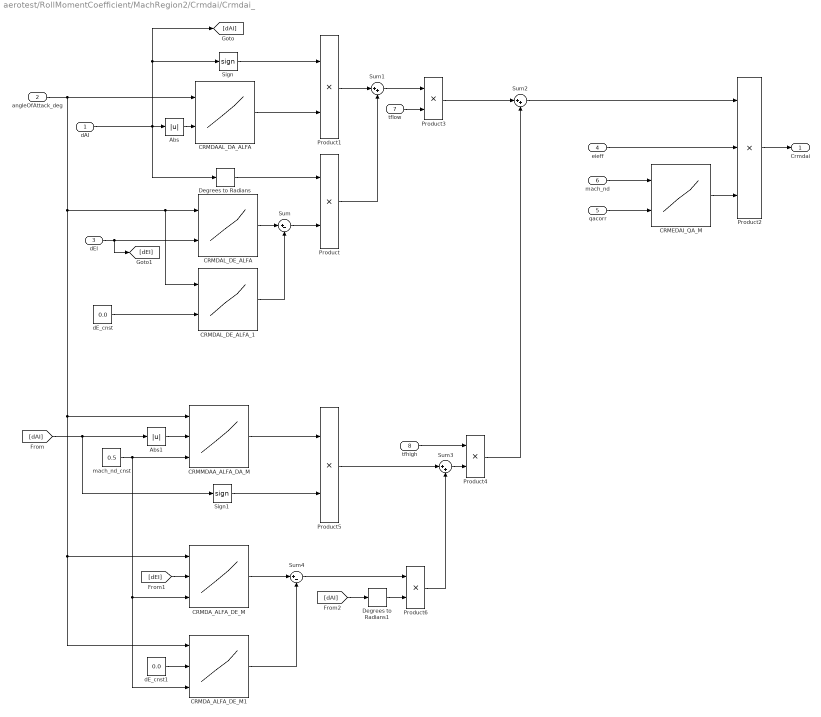
== system aerotest/RollMomentCoefficient/MachRegion2/Crmdai/Crmdai_ ==
  dAI : Inport
  angleOfAttack_deg : Inport  Port=2
  dEI : Inport  Port=3
  eieff : Inport  Port=4
  qacorr : Inport  Port=5
  mach_nd : Inport  Port=6
  tflow : Inport  Port=7
  tfhigh : Inport  Port=8
  Abs : Abs
  Abs1 : Abs
  CRMDAAL_DA_ALFA : Lookup_n-D  BreakpointsForDimension1=admireDB.aerodata_asym_ext.CRMDAAL.breakpoints.ALFA  BreakpointsForDimension2=admireDB.aerodata_asym_ext.CRMDAAL.breakpoints.DA  BreakpointsForDimension3=[5, 7]  Table=admireDB.aerodata_asym_ext.CRMDAAL.newTable  ExtrapMethod=Clip  InternalRulePriority=Speed  RndMeth=Simplest  InputSameDT=on
      settings: InputPortMap=u0,u1
  CRMDAL_DE_ALFA : Lookup_n-D  BreakpointsForDimension1=admireDB.aerodata_asym_ext.CRMDAL.breakpoints.ALFA  BreakpointsForDimension2=admireDB.aerodata_asym_ext.CRMDAL.breakpoints.DE  BreakpointsForDimension3=[5, 7]  Table=admireDB.aerodata_asym_ext.CRMDAL.newTable  ExtrapMethod=Clip  InternalRulePriority=Speed  RndMeth=Simplest  InputSameDT=on
      settings: InputPortMap=u0,u1
  CRMDAL_DE_ALFA_1 : Lookup_n-D  BreakpointsForDimension1=admireDB.aerodata_asym_ext.CRMDAL.breakpoints.ALFA  BreakpointsForDimension2=admireDB.aerodata_asym_ext.CRMDAL.breakpoints.DE  BreakpointsForDimension3=[5, 7]  Table=admireDB.aerodata_asym_ext.CRMDAL.newTable  ExtrapMethod=Clip  InternalRulePriority=Speed  RndMeth=Simplest  InputSameDT=on
      settings: InputPortMap=u0,u1
  CRMDA_ALFA_DE_M : Lookup_n-D  NumberOfTableDimensions=3  BreakpointsForDimension1=admireDB.aerodata_asym_ext.CRMDA.breakpoints.ALFA  BreakpointsForDimension2=admireDB.aerodata_asym_ext.CRMDA.breakpoints.DE  BreakpointsForDimension3=admireDB.aerodata_asym_ext.CRMDA.breakpoints.M  Table=admireDB.aerodata_asym_ext.CRMDA.newTable  ExtrapMethod=Clip  InternalRulePriority=Speed  RndMeth=Simplest  InputSameDT=on
      settings: InputPortMap=u0,u1,u2
  CRMDA_ALFA_DE_M1 : Lookup_n-D  NumberOfTableDimensions=3  BreakpointsForDimension1=admireDB.aerodata_asym_ext.CRMDA.breakpoints.ALFA  BreakpointsForDimension2=admireDB.aerodata_asym_ext.CRMDA.breakpoints.DE  BreakpointsForDimension3=admireDB.aerodata_asym_ext.CRMDA.breakpoints.M  Table=admireDB.aerodata_asym_ext.CRMDA.newTable  ExtrapMethod=Clip  InternalRulePriority=Speed  RndMeth=Simplest  InputSameDT=on
      settings: InputPortMap=u0,u1,u2
  CRMEDAI_QA_M : Lookup_n-D  BreakpointsForDimension1=admireDB.aerodata_asym_ext.CRMEDAI.breakpoints.M  BreakpointsForDimension2=admireDB.aerodata_asym_ext.CRMEDAI.breakpoints.QA  BreakpointsForDimension3=[5, 7]  Table=admireDB.aerodata_asym_ext.CRMEDAI.newTable  ExtrapMethod=Clip  InternalRulePriority=Speed  RndMeth=Simplest  InputSameDT=on
      settings: InputPortMap=u0,u1
  CRMMDAA_ALFA_DA_M : Lookup_n-D  NumberOfTableDimensions=3  BreakpointsForDimension1=admireDB.aerodata_asym_ext.CRMMDAA.breakpoints.ALFA  BreakpointsForDimension2=admireDB.aerodata_asym_ext.CRMMDAA.breakpoints.DA  BreakpointsForDimension3=admireDB.aerodata_asym_ext.CRMMDAA.breakpoints.M  Table=admireDB.aerodata_asym_ext.CRMMDAA.newTable  ExtrapMethod=Clip  InternalRulePriority=Speed  RndMeth=Simplest  InputSameDT=on
      settings: InputPortMap=u0,u1,u2
  Degrees to Radians : simulink_extras/Transformations/Degrees to Radians
  Degrees to Radians1 : simulink_extras/Transformations/Degrees to Radians
  Product{,1,3..4,6} (5 alike) : Product
  Product2 : Product  Inputs=3
  Product5 : Product  Inputs=**
  Sign : Signum
  Sign1 : Signum
  Sum : Sum  Inputs=|+-
  Sum1 : Sum  Inputs=|++
  Sum2 : Sum  Inputs=|++
  Sum3 : Sum  Inputs=|++
  Sum4 : Sum  Inputs=|+-
  dE_cnst : Constant  Value=0.0
  dE_cnst1 : Constant  Value=0.0
  mach_nd_cnst : Constant  Value=0.5
  Crmdai : Outport
  wires:
  Sum3/1 -> Product4/2
  Product6/1 -> Sum3/2
  [dAI] -> Degrees to Radians1/1
  Degrees to Radians1/1 -> Product6/2
  Sum4/1 -> Product6/1
  CRMDA_ALFA_DE_M1/1 -> Sum4/2
  CRMDA_ALFA_DE_M/1 -> Sum4/1
  dE_cnst1/1 -> CRMDA_ALFA_DE_M1/2
  [dEI] -> CRMDA_ALFA_DE_M/2
  mach_nd_cnst/1 -> CRMDA_ALFA_DE_M/3, CRMDA_ALFA_DE_M1/3, CRMMDAA_ALFA_DA_M/3
  Product5/1 -> Sum3/1
  Abs1/1 -> CRMMDAA_ALFA_DA_M/2
  CRMMDAA_ALFA_DA_M/1 -> Product5/1
  [dAI] -> Sign1/1, Abs1/1
  Sign1/1 -> Product5/2
  angleOfAttack_deg/1 -> CRMDAAL_DA_ALFA/1, CRMDAL_DE_ALFA/1, CRMDAL_DE_ALFA_1/1, CRMMDAA_ALFA_DA_M/1, CRMDA_ALFA_DE_M1/1, CRMDA_ALFA_DE_M/1
  Product4/1 -> Sum2/2
  Product3/1 -> Sum2/1
  tfhigh/1 -> Product4/1
  Sum2/1 -> Product2/1
  tflow/1 -> Product3/2
  Product2/1 -> Crmdai/1
  dAI/1 -> Sign/1, [dAI], Abs/1, Degrees to Radians/1
  Abs/1 -> CRMDAAL_DA_ALFA/2
  dE_cnst/1 -> CRMDAL_DE_ALFA_1/2
  dEI/1 -> [dEI], CRMDAL_DE_ALFA/2
  CRMDAL_DE_ALFA/1 -> Sum/1
  CRMDAL_DE_ALFA_1/1 -> Sum/2
  Sum/1 -> Product/2
  Degrees to Radians/1 -> Product/1
  CRMDAAL_DA_ALFA/1 -> Product1/2
  Sign/1 -> Product1/1
  Product1/1 -> Sum1/1
  Product/1 -> Sum1/2
  Sum1/1 -> Product3/1
  eieff/1 -> Product2/2
  qacorr/1 -> CRMEDAI_QA_M/2
  mach_nd/1 -> CRMEDAI_QA_M/1
  CRMEDAI_QA_M/1 -> Product2/3

== system aerotest/RollMomentCoefficient/MachRegion2/Crmdaib/Crmdaib_ ==
  angleOfAttack_deg : Inport
  dAI : Inport  Port=2
  angleOfSideslip_deg : Inport  Port=3
  eieff : Inport  Port=4
  tflow : Inport  Port=5
  Abs : Abs
  Abs1 : Abs
  Abs2 : Abs
  CRMDABAL_ALFA : Lookup_n-D  NumberOfTableDimensions=1  BreakpointsForDimension1=admireDB.aerodata_asym_ext.CRMDABAL.breakpoints.ALFA  BreakpointsForDimension3=[5, 7]  Table=admireDB.aerodata_asym_ext.CRMDABAL.newTable  ExtrapMethod=Clip  InternalRulePriority=Speed  RndMeth=Simplest  InputSameDT=on
  Constant : Constant  Value=1/30
  Constant1 : Constant  Value=1/20
  Product : Product  Inputs=*******
  Crmdaib : Outport
  wires:
  tflow/1 -> Product/7
  Product/1 -> Crmdaib/1
  angleOfAttack_deg/1 -> Abs/1
  CRMDABAL_ALFA/1 -> Product/1
  dAI/1 -> Abs1/1
  Abs/1 -> CRMDABAL_ALFA/1
  Abs1/1 -> Product/2
  Constant/1 -> Product/3
  angleOfSideslip_deg/1 -> Abs2/1
  Constant1/1 -> Product/5
  Abs2/1 -> Product/4
  eieff/1 -> Product/6

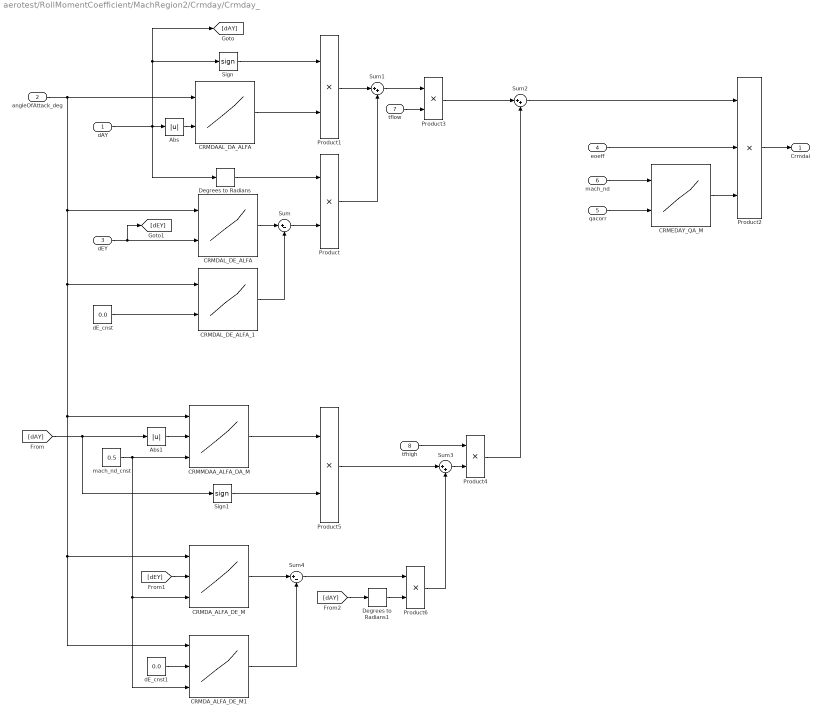
== system aerotest/RollMomentCoefficient/MachRegion2/Crmday/Crmday_ ==
  dAY : Inport
  angleOfAttack_deg : Inport  Port=2
  dEY : Inport  Port=3
  eoeff : Inport  Port=4
  qacorr : Inport  Port=5
  mach_nd : Inport  Port=6
  tflow : Inport  Port=7
  tfhigh : Inport  Port=8
  Abs : Abs
  Abs1 : Abs
  CRMDAAL_DA_ALFA : Lookup_n-D  BreakpointsForDimension1=admireDB.aerodata_asym_ext.CRMDAAL.breakpoints.ALFA  BreakpointsForDimension2=admireDB.aerodata_asym_ext.CRMDAAL.breakpoints.DA  BreakpointsForDimension3=[5, 7]  Table=admireDB.aerodata_asym_ext.CRMDAAL.newTable  ExtrapMethod=Clip  InternalRulePriority=Speed  RndMeth=Simplest  InputSameDT=on
      settings: InputPortMap=u0,u1
  CRMDAL_DE_ALFA : Lookup_n-D  BreakpointsForDimension1=admireDB.aerodata_asym_ext.CRMDAL.breakpoints.ALFA  BreakpointsForDimension2=admireDB.aerodata_asym_ext.CRMDAL.breakpoints.DE  BreakpointsForDimension3=[5, 7]  Table=admireDB.aerodata_asym_ext.CRMDAL.newTable  ExtrapMethod=Clip  InternalRulePriority=Speed  RndMeth=Simplest  InputSameDT=on
      settings: InputPortMap=u0,u1
  CRMDAL_DE_ALFA_1 : Lookup_n-D  BreakpointsForDimension1=admireDB.aerodata_asym_ext.CRMDAL.breakpoints.ALFA  BreakpointsForDimension2=admireDB.aerodata_asym_ext.CRMDAL.breakpoints.DE  BreakpointsForDimension3=[5, 7]  Table=admireDB.aerodata_asym_ext.CRMDAL.newTable  ExtrapMethod=Clip  InternalRulePriority=Speed  RndMeth=Simplest  InputSameDT=on
      settings: InputPortMap=u0,u1
  CRMDA_ALFA_DE_M : Lookup_n-D  NumberOfTableDimensions=3  BreakpointsForDimension1=admireDB.aerodata_asym_ext.CRMDA.breakpoints.ALFA  BreakpointsForDimension2=admireDB.aerodata_asym_ext.CRMDA.breakpoints.DE  BreakpointsForDimension3=admireDB.aerodata_asym_ext.CRMDA.breakpoints.M  Table=admireDB.aerodata_asym_ext.CRMDA.newTable  ExtrapMethod=Clip  InternalRulePriority=Speed  RndMeth=Simplest  InputSameDT=on
      settings: InputPortMap=u0,u1,u2
  CRMDA_ALFA_DE_M1 : Lookup_n-D  NumberOfTableDimensions=3  BreakpointsForDimension1=admireDB.aerodata_asym_ext.CRMDA.breakpoints.ALFA  BreakpointsForDimension2=admireDB.aerodata_asym_ext.CRMDA.breakpoints.DE  BreakpointsForDimension3=admireDB.aerodata_asym_ext.CRMDA.breakpoints.M  Table=admireDB.aerodata_asym_ext.CRMDA.newTable  ExtrapMethod=Clip  InternalRulePriority=Speed  RndMeth=Simplest  InputSameDT=on
      settings: InputPortMap=u0,u1,u2
  CRMEDAY_QA_M : Lookup_n-D  BreakpointsForDimension1=admireDB.aerodata_asym_ext.CRMEDAY.breakpoints.M  BreakpointsForDimension2=admireDB.aerodata_asym_ext.CRMEDAY.breakpoints.QA  BreakpointsForDimension3=[5, 7]  Table=admireDB.aerodata_asym_ext.CRMEDAY.newTable  ExtrapMethod=Clip  InternalRulePriority=Speed  RndMeth=Simplest  InputSameDT=on
      settings: InputPortMap=u0,u1
  CRMMDAA_ALFA_DA_M : Lookup_n-D  NumberOfTableDimensions=3  BreakpointsForDimension1=admireDB.aerodata_asym_ext.CRMMDAA.breakpoints.ALFA  BreakpointsForDimension2=admireDB.aerodata_asym_ext.CRMMDAA.breakpoints.DA  BreakpointsForDimension3=admireDB.aerodata_asym_ext.CRMMDAA.breakpoints.M  Table=admireDB.aerodata_asym_ext.CRMMDAA.newTable  ExtrapMethod=Clip  InternalRulePriority=Speed  RndMeth=Simplest  InputSameDT=on
      settings: InputPortMap=u0,u1,u2
  Degrees to Radians : simulink_extras/Transformations/Degrees to Radians
  Degrees to Radians1 : simulink_extras/Transformations/Degrees to Radians
  Product{,1,3..4,6} (5 alike) : Product
  Product2 : Product  Inputs=3
  Product5 : Product  Inputs=**
  Sign : Signum
  Sign1 : Signum
  Sum : Sum  Inputs=|+-
  Sum1 : Sum  Inputs=|++
  Sum2 : Sum  Inputs=|++
  Sum3 : Sum  Inputs=|++
  Sum4 : Sum  Inputs=|+-
  dE_cnst : Constant  Value=0.0
  dE_cnst1 : Constant  Value=0.0
  mach_nd_cnst : Constant  Value=0.5
  Crmdai : Outport
  wires:
  Sum3/1 -> Product4/2
  Product6/1 -> Sum3/2
  [dAY] -> Degrees to Radians1/1
  Degrees to Radians1/1 -> Product6/2
  Sum4/1 -> Product6/1
  CRMDA_ALFA_DE_M1/1 -> Sum4/2
  CRMDA_ALFA_DE_M/1 -> Sum4/1
  dE_cnst1/1 -> CRMDA_ALFA_DE_M1/2
  [dEY] -> CRMDA_ALFA_DE_M/2
  mach_nd_cnst/1 -> CRMDA_ALFA_DE_M/3, CRMDA_ALFA_DE_M1/3, CRMMDAA_ALFA_DA_M/3
  Product5/1 -> Sum3/1
  Abs1/1 -> CRMMDAA_ALFA_DA_M/2
  CRMMDAA_ALFA_DA_M/1 -> Product5/1
  [dAY] -> Sign1/1, Abs1/1
  Sign1/1 -> Product5/2
  angleOfAttack_deg/1 -> CRMDAAL_DA_ALFA/1, CRMDAL_DE_ALFA/1, CRMMDAA_ALFA_DA_M/1, CRMDA_ALFA_DE_M1/1, CRMDA_ALFA_DE_M/1, CRMDAL_DE_ALFA_1/1
  Product4/1 -> Sum2/2
  Product3/1 -> Sum2/1
  tfhigh/1 -> Product4/1
  Sum2/1 -> Product2/1
  tflow/1 -> Product3/2
  Product2/1 -> Crmdai/1
  dAY/1 -> Sign/1, [dAY], Abs/1, Degrees to Radians/1
  Abs/1 -> CRMDAAL_DA_ALFA/2
  dE_cnst/1 -> CRMDAL_DE_ALFA_1/2
  dEY/1 -> CRMDAL_DE_ALFA/2, [dEY]
  CRMDAL_DE_ALFA/1 -> Sum/1
  CRMDAL_DE_ALFA_1/1 -> Sum/2
  Sum/1 -> Product/2
  Degrees to Radians/1 -> Product/1
  CRMDAAL_DA_ALFA/1 -> Product1/2
  Sign/1 -> Product1/1
  Product1/1 -> Sum1/1
  Product/1 -> Sum1/2
  Sum1/1 -> Product3/1
  eoeff/1 -> Product2/2
  qacorr/1 -> CRMEDAY_QA_M/2
  mach_nd/1 -> CRMEDAY_QA_M/1
  CRMEDAY_QA_M/1 -> Product2/3

== system aerotest/RollMomentCoefficient/MachRegion2/Crmdayb/Crmdayb_ ==
  angleOfAttack_deg : Inport
  dAY : Inport  Port=2
  angleOfSideslip_deg : Inport  Port=3
  eoeff : Inport  Port=4
  tflow : Inport  Port=5
  Abs : Abs
  Abs1 : Abs
  Abs2 : Abs
  CRMDABAL_ALFA : Lookup_n-D  NumberOfTableDimensions=1  BreakpointsForDimension1=admireDB.aerodata_asym_ext.CRMDABAL.breakpoints.ALFA  BreakpointsForDimension3=[5, 7]  Table=admireDB.aerodata_asym_ext.CRMDABAL.newTable  ExtrapMethod=Clip  InternalRulePriority=Speed  RndMeth=Simplest  InputSameDT=on
  Constant : Constant  Value=1/30
  Constant1 : Constant  Value=1/20
  Product : Product  Inputs=*******
  Crmdayb : Outport
  wires:
  tflow/1 -> Product/7
  eoeff/1 -> Product/6
  Abs2/1 -> Product/4
  Constant1/1 -> Product/5
  angleOfSideslip_deg/1 -> Abs2/1
  Constant/1 -> Product/3
  Abs1/1 -> Product/2
  Abs/1 -> CRMDABAL_ALFA/1
  dAY/1 -> Abs1/1
  CRMDABAL_ALFA/1 -> Product/1
  angleOfAttack_deg/1 -> Abs/1
  Product/1 -> Crmdayb/1

== system aerotest/RollMomentCoefficient/MachRegion2/Crmdna/Crmdna_ ==
  dNE : Inport
  angleOfAttack_deg : Inport  Port=2
  tflow : Inport  Port=3
  tfhigh : Inport  Port=4
  dNA : Inport  Port=5
  CRMDNAAL_DNE_ALFA : Lookup_n-D  BreakpointsForDimension1=admireDB.aerodata_asym_ext.CRMDNAAL.breakpoints.ALFA  BreakpointsForDimension2=admireDB.aerodata_asym_ext.CRMDNAAL.breakpoints.DNE  BreakpointsForDimension3=[5, 7]  Table=admireDB.aerodata_asym_ext.CRMDNAAL.newTable  ExtrapMethod=Clip  InternalRulePriority=Speed  RndMeth=Simplest  InputSameDT=on
      settings: InputPortMap=u0,u1
  CRMDNAAM_ALFA_M : Lookup_n-D  BreakpointsForDimension1=admireDB.aerodata_asym_ext.CRMDNAAM.breakpoints.M  BreakpointsForDimension2=admireDB.aerodata_asym_ext.CRMDNAAM.breakpoints.ALFA  BreakpointsForDimension3=[5, 7]  Table=admireDB.aerodata_asym_ext.CRMDNAAM.newTable  ExtrapMethod=Clip  InternalRulePriority=Speed  RndMeth=Simplest  InputSameDT=on
      settings: InputPortMap=u0,u1
  Degrees to Radians : simulink_extras/Transformations/Degrees to Radians
  Product : Product  Inputs=**
  Product1 : Product
  Product2 : Product  Inputs=**
  Sum : Sum  Inputs=|++
  mach_nd_cnst : Constant  Value=0.5
  Crmdna : Outport
  wires:
  Sum/1 -> Product/1
  Product2/1 -> Sum/2
  Product1/1 -> Sum/1
  CRMDNAAM_ALFA_M/1 -> Product2/1
  tfhigh/1 -> Product2/2
  mach_nd_cnst/1 -> CRMDNAAM_ALFA_M/1
  tflow/1 -> Product1/2
  Product/1 -> Crmdna/1
  angleOfAttack_deg/1 -> CRMDNAAL_DNE_ALFA/1, CRMDNAAM_ALFA_M/2
  dNE/1 -> CRMDNAAL_DNE_ALFA/2
  dNA/1 -> Degrees to Radians/1
  CRMDNAAL_DNE_ALFA/1 -> Product1/1
  Degrees to Radians/1 -> Product/2

== system aerotest/RollMomentCoefficient/MachRegion2/Crmdr/Crmdr_ ==
  angleOfAttack_deg : Inport
  dR : Inport  Port=2
  tfhigh : Inport  Port=3
  angleOfSideslip_deg : Inport  Port=4
  tflow : Inport  Port=5
  qacorr : Inport  Port=6
  mach_nd : Inport  Port=7
  Abs : Abs
  CRMBDRAL_ALFA_DR_BETA : Lookup_n-D  NumberOfTableDimensions=3  BreakpointsForDimension1=admireDB.aerodata_asym_ext.CRMBDRAL.breakpoints.ALFA  BreakpointsForDimension2=admireDB.aerodata_asym_ext.CRMBDRAL.breakpoints.DR  BreakpointsForDimension3=admireDB.aerodata_asym_ext.CRMBDRAL.breakpoints.BETA  Table=admireDB.aerodata_asym_ext.CRMBDRAL.newTable  ExtrapMethod=Clip  InternalRulePriority=Speed  RndMeth=Simplest  InputSameDT=on
      settings: InputPortMap=u0,u1,u2
  CRMDRM_M : Lookup_n-D  NumberOfTableDimensions=1  BreakpointsForDimension1=admireDB.aerodata_asym_ext.CRMDRM.breakpoints.M  BreakpointsForDimension3=[5, 7]  Table=admireDB.aerodata_asym_ext.CRMDRM.newTable  ExtrapMethod=Clip  InternalRulePriority=Speed  RndMeth=Simplest  InputSameDT=on
  CRMEDR_QA_M : Lookup_n-D  BreakpointsForDimension1=admireDB.aerodata_asym_ext.CRMEDR.breakpoints.M  BreakpointsForDimension2=admireDB.aerodata_asym_ext.CRMEDR.breakpoints.QA  BreakpointsForDimension3=[5, 7]  Table=admireDB.aerodata_asym_ext.CRMEDR.newTable  ExtrapMethod=Clip  InternalRulePriority=Speed  RndMeth=Simplest  InputSameDT=on
      settings: InputPortMap=u0,u1
  Degrees to Radians : simulink_extras/Transformations/Degrees to Radians
  Product : Product
  Product1 : Product  Inputs=***
  Product2 : Product
  Sum : Sum  Inputs=++|
  mach_nd_cnst : Constant  Value=0.5
  Crmdr : Outport
  wires:
  Abs/1 -> CRMBDRAL_ALFA_DR_BETA/3
  Product2/1 -> Crmdr/1
  CRMEDR_QA_M/1 -> Product2/2
  Sum/1 -> Product2/1
  Product1/1 -> Sum/2
  CRMDRM_M/1 -> Product1/1
  Degrees to Radians/1 -> Product1/2
  mach_nd_cnst/1 -> CRMDRM_M/1
  tfhigh/1 -> Product1/3
  dR/1 -> Degrees to Radians/1, CRMBDRAL_ALFA_DR_BETA/2
  Product/1 -> Sum/1
  qacorr/1 -> CRMEDR_QA_M/2
  mach_nd/1 -> CRMEDR_QA_M/1
  angleOfSideslip_deg/1 -> Abs/1
  angleOfAttack_deg/1 -> CRMBDRAL_ALFA_DR_BETA/1
  tflow/1 -> Product/2
  CRMBDRAL_ALFA_DR_BETA/1 -> Product/1

== system aerotest/RollMomentCoefficient/MachRegion2/Crmp/Crmp_ ==
  dN : Inport
  angleOfAttack_deg : Inport  Port=2
  qacorr : Inport  Port=3
  mach_nd : Inport  Port=4
  pc : Inport  Port=5
  tflow : Inport  Port=6
  tfhigh : Inport  Port=7
  CRMEP_QA_M : Lookup_n-D  BreakpointsForDimension1=admireDB.aerodata_asym_ext.CRMEP.breakpoints.M  BreakpointsForDimension2=admireDB.aerodata_asym_ext.CRMEP.breakpoints.QA  BreakpointsForDimension3=[5, 7]  Table=admireDB.aerodata_asym_ext.CRMEP.newTable  ExtrapMethod=Clip  InternalRulePriority=Speed  RndMeth=Simplest  InputSameDT=on
      settings: InputPortMap=u0,u1
  CRMPAL_DN_ALFA : Lookup_n-D  BreakpointsForDimension1=admireDB.aerodata_asym_ext.CRMPAL.breakpoints.ALFA  BreakpointsForDimension2=admireDB.aerodata_asym_ext.CRMPAL.breakpoints.DN  BreakpointsForDimension3=[5, 7]  Table=admireDB.aerodata_asym_ext.CRMPAL.newTable  ExtrapMethod=Clip  InternalRulePriority=Speed  RndMeth=Simplest  InputSameDT=on
      settings: InputPortMap=u0,u1
  CRMPAM_ALFA_M : Lookup_n-D  BreakpointsForDimension1=admireDB.aerodata_asym_ext.CRMPAM.breakpoints.M  BreakpointsForDimension2=admireDB.aerodata_asym_ext.CRMPAM.breakpoints.ALFA  BreakpointsForDimension3=[5, 7]  Table=admireDB.aerodata_asym_ext.CRMPAM.newTable  ExtrapMethod=Clip  InternalRulePriority=Speed  RndMeth=Simplest  InputSameDT=on
      settings: InputPortMap=u0,u1
  Product : Product  Inputs=3
  Product1 : Product  Inputs=**
  Product2 : Product  Inputs=**
  Sum : Sum  Inputs=|++
  mach_nd_cnst : Constant  Value=0.5
  Crmp : Outport
  wires:
  Sum/1 -> Product/1
  Product2/1 -> Sum/2
  Product1/1 -> Sum/1
  tfhigh/1 -> Product2/1
  CRMPAM_ALFA_M/1 -> Product2/2
  tflow/1 -> Product1/2
  mach_nd_cnst/1 -> CRMPAM_ALFA_M/1
  qacorr/1 -> CRMEP_QA_M/2
  mach_nd/1 -> CRMEP_QA_M/1
  angleOfAttack_deg/1 -> CRMPAL_DN_ALFA/1, CRMPAM_ALFA_M/2
  dN/1 -> CRMPAL_DN_ALFA/2
  CRMPAL_DN_ALFA/1 -> Product1/1
  CRMEP_QA_M/1 -> Product/3
  pc/1 -> Product/2
  Product/1 -> Crmp/1
